simulink model "MRAC_Indirect"  (R2016b)
settings: Solver=VariableStepAuto  StartTime=0.0  StopTime=20  RelTol=1e-3
undefined symbols (not defined in the file or in its folder): sigbuilder_block
settings Model: Creator=Niels  LastModifiedBy=Niels

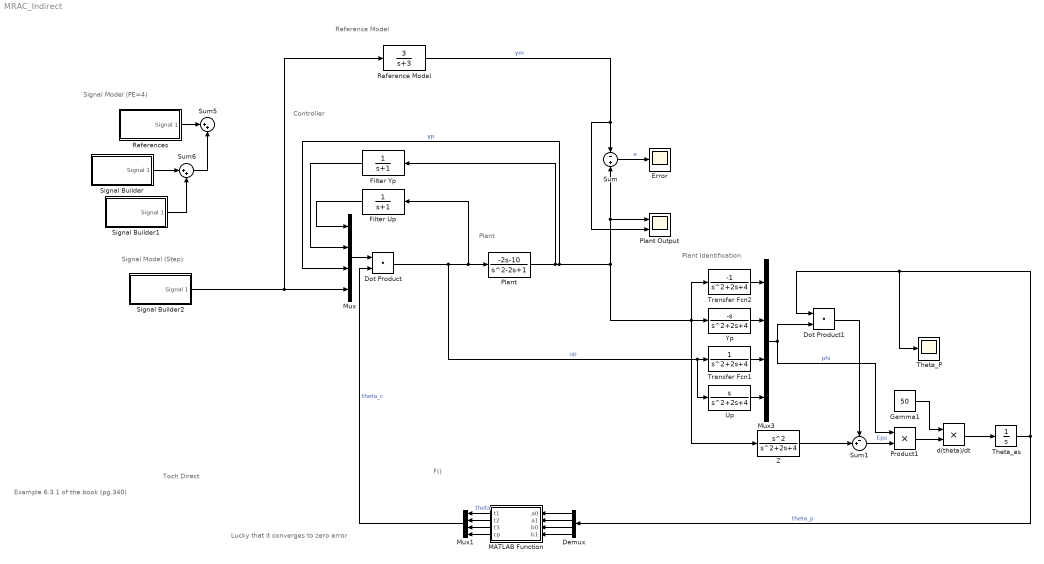
== system MRAC_Indirect ==
  note: Lucky that it converges to zero error
  note: Toch Direct
  note: Signal Model (Step)
  note: Signal Model (PE=4)
  note: F()
  note: Plant
  note: Controller
  note: Reference Model
  note: Plant Identification
  note: Example 6.3.1 of the book (pg.340)
  Demux : Demux
  Dot Product : DotProduct  InputSameDT=on  OutDataTypeStr=Inherit: Inherit via internal rule
  Dot Product1 : DotProduct  InputSameDT=on  OutDataTypeStr=Inherit: Inherit via internal rule
  Error : Scope
  Filter Up : TransferFcn  Denominator=[1 1]
  Filter Yp : TransferFcn  Denominator=[1 1]
  Gamma1 : Constant  Value=50
  MATLAB Function : MATLAB Function  TreatAsAtomicUnit=on
  Mux : Mux
  Mux1 : Mux
  Mux3 : Mux
  Plant : TransferFcn  Numerator=[-2 -10]  Denominator=[1 -2 1]
  Plant Output : Scope  NumInputPorts=2
  Product1 : Product
  Reference Model : TransferFcn  Numerator=[3]  Denominator=[1 3]
  References : Subsystem  Tag=STV Subsys  LoadFcn=sigbuilder_block('load');  StartFcn=sigbuilder_block('start');  StopFcn=sigbuilder_block('stop');  ClipboardFcn=sigbuilder_block('clipboard');  mask(Sigbuilder block){tuvar=[0:10]}
      mask help: Simulink:masks:SigbuilderBlock_MD
      mask init:
      | if ~strcmp(get_param(bdroot(gcbh),'SimulationStatus'),'stopped') tuvar = sigbuilder_block('maskInit'); end
      settings: CopyFcn=sigbuilder_block('copy');  DeleteFcn=sigbuilder_block('delete');  ModelCloseFcn=sigbuilder_block('modelClose');  PreSaveFcn=sigbuilder_block('preSave');  PauseFcn=sigbuilder_block('pause');  ContinueFcn=sigbuilder_block('continue');  NameChangeFcn=sigbuilder_block('namechange');  OpenFcn=sigbuilder_block('open',[437.6 199.2 550.4 400 ]);  CloseFcn=sigbuilder_block('close');
      mask Display: plot(0, 0, 100, 100,[2, 2, 32, 32, 2], [68, 8, 8, 68, 68],[32, 2], [38, 38], [32, 19, 2],[53, 60, 44], [32, 17, 17, 2],[16, 16, 31, 31]);txt = getActiveGroup(gcbh);text(2, 100, txt,'verticalAlignment', 'top');
  Signal Builder : Subsystem  Tag=STV Subsys  LoadFcn=sigbuilder_block('load');  StartFcn=sigbuilder_block('start');  StopFcn=sigbuilder_block('stop');  ClipboardFcn=sigbuilder_block('clipboard');  mask(Sigbuilder block){tuvar=[0:10]}
      mask help: Simulink:masks:SigbuilderBlock_MD
      mask init:
      | if ~strcmp(get_param(bdroot(gcbh),'SimulationStatus'),'stopped') tuvar = sigbuilder_block('maskInit'); end
      settings: CopyFcn=sigbuilder_block('copy');  DeleteFcn=sigbuilder_block('delete');  ModelCloseFcn=sigbuilder_block('modelClose');  PreSaveFcn=sigbuilder_block('preSave');  PauseFcn=sigbuilder_block('pause');  ContinueFcn=sigbuilder_block('continue');  NameChangeFcn=sigbuilder_block('namechange');  OpenFcn=sigbuilder_block('open',[437.6 199.2 550.4 400 ]);  CloseFcn=sigbuilder_block('close');
      mask Display: plot(0, 0, 100, 100,[2, 2, 32, 32, 2], [68, 8, 8, 68, 68],[32, 2], [38, 38], [32, 19, 2],[53, 60, 44], [32, 17, 17, 2],[16, 16, 31, 31]);txt = getActiveGroup(gcbh);text(2, 100, txt,'verticalAlignment', 'top');
  Signal Builder1 : Subsystem  Tag=STV Subsys  LoadFcn=sigbuilder_block('load');  StartFcn=sigbuilder_block('start');  StopFcn=sigbuilder_block('stop');  ClipboardFcn=sigbuilder_block('clipboard');  mask(Sigbuilder block){tuvar=[0:10]}
      mask help: Simulink:masks:SigbuilderBlock_MD
      mask init:
      | if ~strcmp(get_param(bdroot(gcbh),'SimulationStatus'),'stopped') tuvar = sigbuilder_block('maskInit'); end
      settings: CopyFcn=sigbuilder_block('copy');  DeleteFcn=sigbuilder_block('delete');  ModelCloseFcn=sigbuilder_block('modelClose');  PreSaveFcn=sigbuilder_block('preSave');  PauseFcn=sigbuilder_block('pause');  ContinueFcn=sigbuilder_block('continue');  NameChangeFcn=sigbuilder_block('namechange');  OpenFcn=sigbuilder_block('open',[437.6 199.2 550.4 400 ]);  CloseFcn=sigbuilder_block('close');
      mask Display: plot(0, 0, 100, 100,[2, 2, 32, 32, 2], [68, 8, 8, 68, 68],[32, 2], [38, 38], [32, 19, 2],[53, 60, 44], [32, 17, 17, 2],[16, 16, 31, 31]);txt = getActiveGroup(gcbh);text(2, 100, txt,'verticalAlignment', 'top');
  Signal Builder2 : Subsystem  Tag=STV Subsys  LoadFcn=sigbuilder_block('load');  StartFcn=sigbuilder_block('start');  StopFcn=sigbuilder_block('stop');  ClipboardFcn=sigbuilder_block('clipboard');  mask(Sigbuilder block){tuvar=[0:10]}
      mask help: Simulink:masks:SigbuilderBlock_MD
      mask init:
      | if ~strcmp(get_param(bdroot(gcbh),'SimulationStatus'),'stopped') tuvar = sigbuilder_block('maskInit'); end
      settings: CopyFcn=sigbuilder_block('copy');  DeleteFcn=sigbuilder_block('delete');  ModelCloseFcn=sigbuilder_block('modelClose');  PreSaveFcn=sigbuilder_block('preSave');  PauseFcn=sigbuilder_block('pause');  ContinueFcn=sigbuilder_block('continue');  NameChangeFcn=sigbuilder_block('namechange');  OpenFcn=sigbuilder_block('open',[437.6 199.2 550.4 400 ]);  CloseFcn=sigbuilder_block('close');
      mask Display: plot(0, 0, 100, 100,[2, 2, 32, 32, 2], [68, 8, 8, 68, 68],[32, 2], [38, 38], [32, 19, 2],[53, 60, 44], [32, 17, 17, 2],[16, 16, 31, 31]);txt = getActiveGroup(gcbh);text(2, 100, txt,'verticalAlignment', 'top');
  Sum : Sum  Inputs=-|+
  Sum1 : Sum  Inputs=-+|
  Sum5 : Sum  Inputs=|++
  Sum6 : Sum  Inputs=|++
  Theta_P : Scope
  Theta_es : Integrator  InitialCondition=[1;1;1;1]
  Transfer Fcn1 : TransferFcn  Denominator=[1 2 4]
  Transfer Fcn2 : TransferFcn  Numerator=[-1]  Denominator=[1 2 4]
  Up : TransferFcn  Numerator=[1 0]  Denominator=[1 2 4]
  Yp : TransferFcn  Numerator=[-1 0]  Denominator=[1 2 4]
  Z : TransferFcn  Numerator=[1 0 0]  Denominator=[1 2 4]
  d(theta)/dt : Product
  wires:
  Mux/1 -> Dot Product/1
  Dot Product/1 -> Up/1, Transfer Fcn1/1, Plant/1, Filter Up/1  "up"
  Filter Up/1 -> Mux/1
  Plant/1 -> Z/1, Transfer Fcn2/1, Yp/1, Sum/2, Plant Output/1, Mux/3, Filter Yp/1  "yp"
  Reference Model/1 -> Plant Output/2, Sum/1  "ym"
  Filter Yp/1 -> Mux/2
  Sum/1 -> Error/1  "e"
  MATLAB Function/4(cp) -> Mux1/4
  MATLAB Function/3(t3) -> Mux1/3
  MATLAB Function/2(t2) -> Mux1/2
  MATLAB Function/1(t1) -> Mux1/1  "theta"
  Mux1/1 -> Dot Product/2  "theta_c"
  Up/1 -> Mux3/4
  Yp/1 -> Mux3/2
  Mux3/1 -> Dot Product1/2, Product1/1  "phi"
  Theta_es/1 -> Demux/1, Theta_P/1, Dot Product1/1  "theta_p"
  Z/1 -> Sum1/2
  Dot Product1/1 -> Sum1/1
  Sum1/1 -> Product1/2  "Eps"
  Gamma1/1 -> d(theta)/dt/1
  d(theta)/dt/1 -> Theta_es/1
  Product1/1 -> d(theta)/dt/2
  Transfer Fcn2/1 -> Mux3/1
  Transfer Fcn1/1 -> Mux3/3
  References/1(Signal 1) -> Sum5/1
  Sum6/1 -> Sum5/2
  Signal Builder/1(Signal 1) -> Sum6/1
  Signal Builder1/1(Signal 1) -> Sum6/2
  Demux/1 -> MATLAB Function/1(a0)
  Demux/2 -> MATLAB Function/2(a1)
  Demux/3 -> MATLAB Function/3(b0)
  Demux/4 -> MATLAB Function/4(b1)
  Signal Builder2/1(Signal 1) -> Reference Model/1, Mux/4

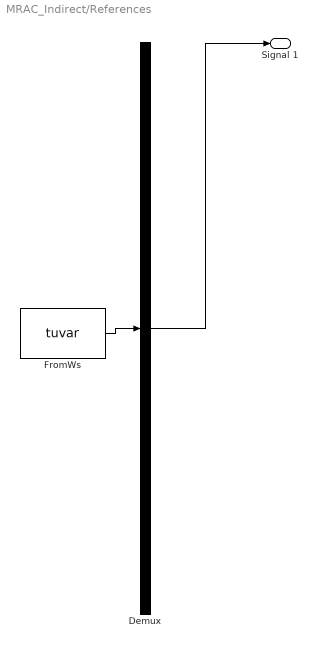
== system MRAC_Indirect/References ==
  Demux : Demux  Tag=STV Demux  Outputs=1
  FromWs : FromWorkspace  Tag=STV FromWs  VariableName=tuvar  SampleTime=0
      SigBuilderData=|
      | common.afterFinalStr = 'Extrapolate'
      | common.sampleTime = 0
      | dataSet.timeRange = [0 6000]
      | dataSet.name = 'Group 1'
      | sbobj.Groups.Name = 'Group 1'
      | sbobj.Groups.Signals.Name = 'Signal 1'
      | sbobj.Groups.Signals.XData = [0 0.125 0.25 0.375 0.5 0.625 0.75 0.875 1 1.125 1.25 1.375 ... (40005 elements, 1x40005)]
      | sbobj.Groups.Signals.YData = [1 1.70710678119 2 1.70710678119 1 0.292893218813 0 0.292893218813 1 1.70710678119 2 1.70710678119 ... (40005 elements, 1x40005)]
      | sbobj.Groups.TimeRange = [0 6000]
  Signal 1 : Outport  Tag=STV Outport
  wires:
  Demux/1 -> Signal 1/1
  FromWs/1 -> Demux/1

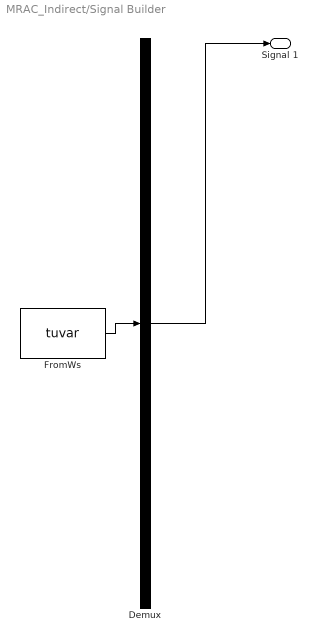
== system MRAC_Indirect/Signal Builder ==
  Demux : Demux  Tag=STV Demux  Outputs=1
  FromWs : FromWorkspace  Tag=STV FromWs  VariableName=tuvar  SampleTime=0
      SigBuilderData=|
      | common.afterFinalStr = 'Extrapolate'
      | common.sampleTime = 0
      | dataSet.timeRange = [0 5000]
      | dataSet.name = 'Group 1'
      | sbobj.Groups.Name = 'Group 1'
      | sbobj.Groups.Signals.Name = 'Signal 1'
      | sbobj.Groups.Signals.XData = [0 0.0166666666667 0.0333333333333 0.05 0.0666666666667 0.0833333333333 0.1 0.116666666667 0.133333333333 0.15 0.166666666667 0.183333333333 ... (300001 elements, 1x300001)]
      | sbobj.Groups.Signals.YData = [1 1.70710678119 2 1.70710678119 1 0.292893218813 0 0.292893218813 1 1.70710678119 2 1.70710678119 ... (300001 elements, 1x300001)]
      | sbobj.Groups.TimeRange = [0 5000]
  Signal 1 : Outport  Tag=STV Outport
  wires:
  Demux/1 -> Signal 1/1
  FromWs/1 -> Demux/1

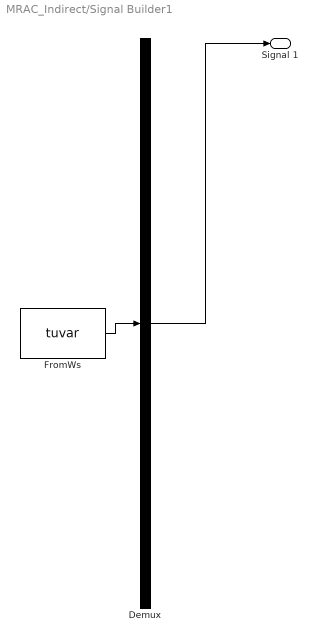
== system MRAC_Indirect/Signal Builder1 ==
  Demux : Demux  Tag=STV Demux  Outputs=1
  FromWs : FromWorkspace  Tag=STV FromWs  VariableName=tuvar  SampleTime=0
      SigBuilderData=|
      | common.afterFinalStr = 'Extrapolate'
      | common.sampleTime = 0
      | dataSet.timeRange = [0 5000]
      | dataSet.name = 'Group 1'
      | sbobj.Groups.Name = 'Group 1'
      | sbobj.Groups.Signals.Name = 'Signal 1'
      | sbobj.Groups.Signals.XData = [0 0.416666666667 0.833333333333 1.25 1.66666666667 2.08333333333 2.5 2.91666666667 3.33333333333 3.75 4.16666666667 4.58333333333 ... (12001 elements, 1x12001)]
      | sbobj.Groups.Signals.YData = [1 1.70710678119 2 1.70710678119 1 0.292893218813 0 0.292893218813 1 1.70710678119 2 1.70710678119 ... (12001 elements, 1x12001)]
      | sbobj.Groups.TimeRange = [0 5000]
  Signal 1 : Outport  Tag=STV Outport
  wires:
  Demux/1 -> Signal 1/1
  FromWs/1 -> Demux/1

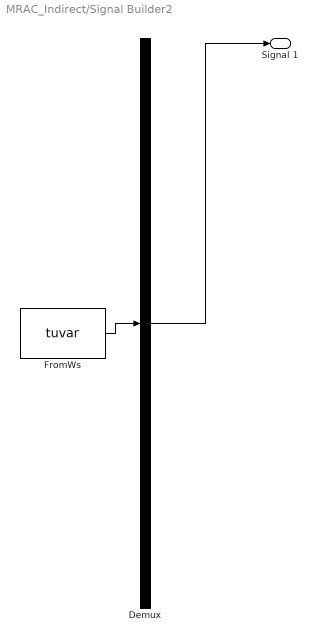
== system MRAC_Indirect/Signal Builder2 ==
  Demux : Demux  Tag=STV Demux  Outputs=1
  FromWs : FromWorkspace  Tag=STV FromWs  VariableName=tuvar  SampleTime=0
      SigBuilderData=|
      | common.afterFinalStr = 'Extrapolate'
      | common.sampleTime = 0
      | dataSet.timeRange = [0 10]
      | dataSet.name = 'Group 1'
      | sbobj.Groups.Name = 'Group 1'
      | sbobj.Groups.Signals.Name = 'Signal 1'
      | sbobj.Groups.Signals.XData = [0 1.1 1.1 6 6 10]
      | sbobj.Groups.Signals.YData = [0 0 1 1 1.99 1.99]
  Signal 1 : Outport  Tag=STV Outport
  wires:
  Demux/1 -> Signal 1/1
  FromWs/1 -> Demux/1

== matlab function MRAC_Indirect/MATLAB Function ==
  data: t1 output; t2 output; t3 output; cp output; a0 input; a1 input; b0 input; b1 input
function [t1,t2,t3,cp] = F(a0,a1,b0,b1)
cp = 3/b1;
A = [1 0 b1; a1 b1 b1+b0; a0 b0 b0];
b = [a1-b0/b1-3; a1+a0-3-4*b0/b1; a0-3*b0/b1];
T = A\b;
t1 = T(1);
t2 = T(2);
t3 = T(3);
end
